simulink library "calcLogLikelihood_ul"  (R2018b)
settings: Solver=VariableStepAuto  StartTime=0.0  StopTime=10.0  RelTol=1e-3
libraries: buildSqrdExpCovMat_ul x1
settings Model: Creator=asiddiq2  LastModifiedBy=asiddiq2

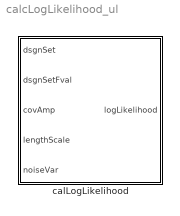
== system calcLogLikelihood_ul ==
  calLogLikelihood : Subsystem

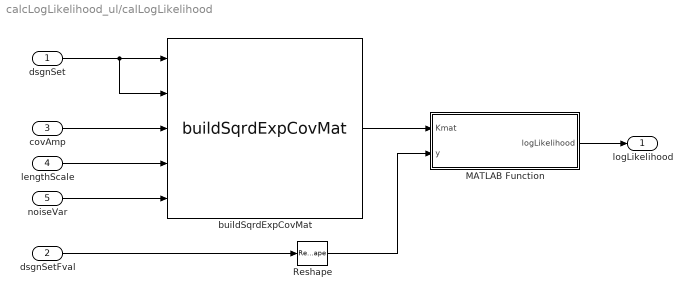
== system calcLogLikelihood_ul/calLogLikelihood ==
  dsgnSet : Inport
  dsgnSetFval : Inport  Port=2
  covAmp : Inport  Port=3
  lengthScale : Inport  Port=4
  noiseVar : Inport  Port=5
  MATLAB Function : MATLAB Function  TreatAsAtomicUnit=on
  Reshape : Reshape  OutputDimensionality=Column vector (2-D)
  buildSqrdExpCovMat : buildSqrdExpCovMat_ul/buildSqrdExpCovMat  SystemSampleTime=-1
  logLikelihood : Outport
  wires:
  lengthScale/1 -> buildSqrdExpCovMat/4
  buildSqrdExpCovMat/1 -> MATLAB Function/1(Kmat)
  MATLAB Function/1(logLikelihood) -> logLikelihood/1
  dsgnSet/1 -> buildSqrdExpCovMat/2, buildSqrdExpCovMat/1
  covAmp/1 -> buildSqrdExpCovMat/3
  noiseVar/1 -> buildSqrdExpCovMat/5
  dsgnSetFval/1 -> Reshape/1
  Reshape/1 -> MATLAB Function/2(y)

== matlab function calcLogLikelihood_ul/calLogLikelihood/MATLAB Function ==
  data: Kmat input; logLikelihood output; y input
function logLikelihood = fcn(Kmat,y)

logLikelihood = 1*(-0.5*(y'/Kmat*y) - 0.5*log(det(Kmat)));

end
